simulink model "stateflow_uniqueStatename"  (R2016b)
settings: Solver=FixedStepDiscrete  StartTime=0.0  StopTime=inf  RelTol=1e-3  EnableMultiTasking=on
settings Model: Creator=amyyang  LastModifiedBy=amyyang
settings DataIOCC: LimitDataPoints=on
settings OptimizationCC: DefaultParameterBehavior=Inlined  LifeSpan=1
settings DebuggingCC: AllowSymbolicDim=off  SFUnexpectedBacktrackingDiag=warning  SFNoUnconditionalDefaultTransitionDiag=warning  SFExecutionAtInitializationDiag=none
settings ModelReferenceCC: PropagateSignalLabelsOutOfModel=off
settings RTWCC: SystemTargetFile=ert.tlc  GenCodeOnly=on  TemplateMakefile=ert_default_tmf  Description=Embedded Coder  GenerateReport=on  IncludeHyperlinkInReport=on  LaunchReport=on  GenerateTraceInfo=on  GenerateTraceReport=on  GenerateTraceReportSl=on  GenerateTraceReportSf=on  GenerateTraceReportEml=on
settings CodeAppCC: IgnoreCustomStorageClasses=off
settings ERTTargetCC: GenerateSampleERTMain=on  InlinedParameterPlacement=NonHierarchical  ERTCustomFileTemplate=example_file_process.tlc  ConvertIfToSwitch=off  SuppressUnreachableDefaultCases=off
settings ConfigComp: CovMetricSettings=dw  CovHtmlReporting=on  CovSaveCumulativeToWorkspaceVar=on  CovSaveSingleToWorkspaceVar=on  CovExternalEMLEnable=off

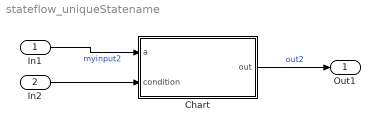
== system stateflow_uniqueStatename ==
  In1 : Inport
  In2 : Inport  Port=2
  Chart : Stateflow chart  TreatAsAtomicUnit=on
  Out1 : Outport
  wires:
  Chart/1(out) -> Out1/1  "out2"
  In1/1 -> Chart/1(a)  "myinput2"
  In2/1 -> Chart/2(condition)

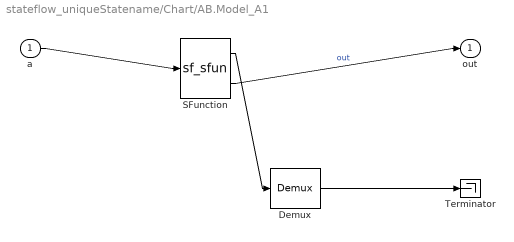
== system stateflow_uniqueStatename/Chart/AB.Model_A1 ==
  a : Inport
  " Demux " : Demux  Outputs=1
  " SFunction " : S-Function  Tag=Stateflow S-Function stateflow_uniqueStatename 1  FunctionName=sf_sfun  PortCounts=[1 2]  SFunctionDeploymentMode=off  EnableBusSupport=off
  " Terminator " : Terminator
  out : Outport
  wires:
  a/1 -> " SFunction "/1
  " SFunction "/2 -> out/1  "out"
  " Demux "/1 -> " Terminator "/1
  " SFunction "/1 -> " Demux "/1

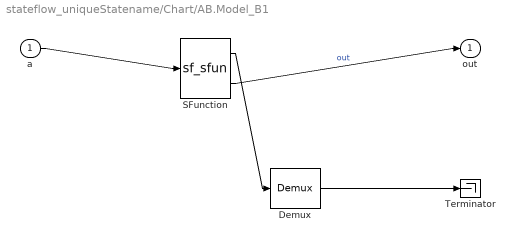
== system stateflow_uniqueStatename/Chart/AB.Model_B1 ==
  a : Inport
  " Demux " : Demux  Outputs=1
  " SFunction " : S-Function  Tag=Stateflow S-Function stateflow_uniqueStatename 2  FunctionName=sf_sfun  PortCounts=[1 2]  SFunctionDeploymentMode=off  EnableBusSupport=off
  " Terminator " : Terminator
  out : Outport
  wires:
  a/1 -> " SFunction "/1
  " SFunction "/2 -> out/1  "out"
  " Demux "/1 -> " Terminator "/1
  " SFunction "/1 -> " Demux "/1

== stateflow chart stateflow_uniqueStatename/Chart/AB.Model_A1 ==
  state Off_A
    en:
    out = 1;
  state On_A
    en:
    out = 2;
  (default) -> Off_A
  Off_A -> On_A : [a]
  On_A -> Off_A : [~a]
  data: a input; out output

== stateflow chart stateflow_uniqueStatename/Chart/AB.Model_B1 ==
  state Off_A
    en:
    out = 1;
  state On_A
    en:
    out = 2;
  (default) -> Off_A
  Off_A -> On_A : [a]
  On_A -> Off_A : [~a]
  data: a input; out output

== stateflow chart stateflow_uniqueStatename/Chart ==
  state AA [parallel]
    settings: executionOrder=1
    state Model_B
      state Off_A
        en:
        out = 3;
      state On_B
        en:
        out = 4;
      (default) -> AA.Model_B.Off_A
      AA.Model_B.Off_A -> On_B : [a]
      On_B -> AA.Model_B.Off_A : [~a]
    state Model_A
      state Off_A
        en:
        out = 1;
      state On_A
        en:
        out = 2;
      (default) -> AA.Model_A.Off_A
      AA.Model_A.Off_A -> On_A : [a]
      On_A -> AA.Model_A.Off_A : [~a]
    (default) -> Model_A
    Model_A -> Model_B : [ condition]
    Model_B -> Model_A : [ condition]
  state AB [parallel]
    settings: executionOrder=2
    state Model_B1
    state Model_A1
    (default) -> Model_A1
    Model_A1 -> Model_B1 : [ condition]
    Model_B1 -> Model_A1 : [ condition]
  data: out output; a input; data local; condition input
